simulink model "pll"  (Simulink 7.2)
settings: Solver=ode3  StartTime=0.0  StopTime=1  FixedStep=1e-5  RelTol=1e-3
libraries: dsparch4 x1, commsynccomp2 x1
settings Model: Creator=OTHMANE  LastModifiedBy=OTHMANE

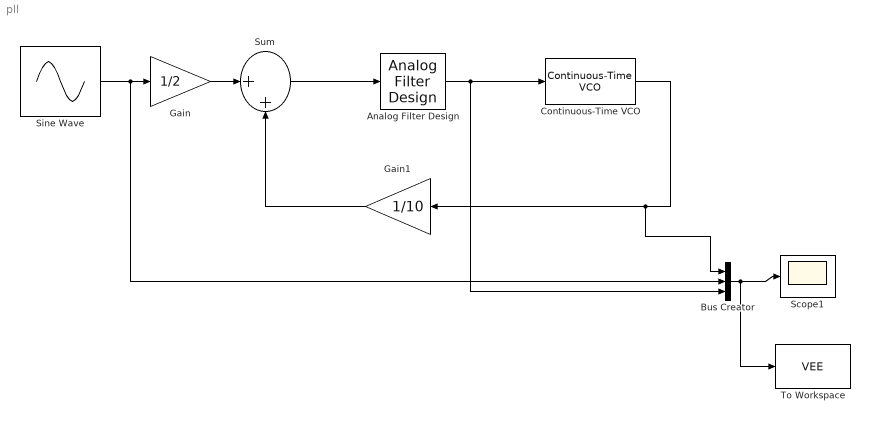
== system pll ==
  Analog Filter Design : dsparch4/Analog Filter Design  method=Butterworth  filttype=Lowpass  N=1  Wlo=100  Whi=80  Rp=2  Rs=40
  Bus Creator : BusCreator  Inputs=3
  Continuous-Time VCO : commsynccomp2/Continuous-Time VCO  SystemSampleTime=-1  Ac=1  Fc=10  Kc=1  Ph=0
  Gain : Gain  Gain=1/2  ParameterDataType=sfix(16)  ParameterScaling=2^0  OutDataType=sfix(16)  OutScaling=2^0
  Gain1 : Gain  Orientation=left  Gain=1/10  ParameterDataType=sfix(16)  ParameterScaling=2^0  OutDataType=sfix(16)  OutScaling=2^0
  Scope1 : Scope
      settings: YMin=-3  YMax=3
  Sine Wave : Sin  Frequency=50  SampleTime=0
  Sum : Sum  Inputs=|++  OutDataType=sfix(16)  OutScaling=2^0
  To Workspace : ToWorkspace  VariableName=VEE  SampleTime=-1  SaveFormat=Array
  wires:
  Continuous-Time VCO/1 -> Gain1/1, Bus Creator/1
  Bus Creator/1 -> Scope1/1, To Workspace/1
  Sum/1 -> Analog Filter Design/1
  Analog Filter Design/1 -> Continuous-Time VCO/1, Bus Creator/3
  Gain/1 -> Sum/1
  Sine Wave/1 -> Gain/1, Bus Creator/2
  Gain1/1 -> Sum/2
